simulink model "Lab_1_Part_1_6"  (R2019b)
settings: Solver=VariableStepAuto  StartTime=0.0  StopTime=10.0  RelTol=1e-3
settings Model: Creator=mikewang  LastModifiedBy=mikewang

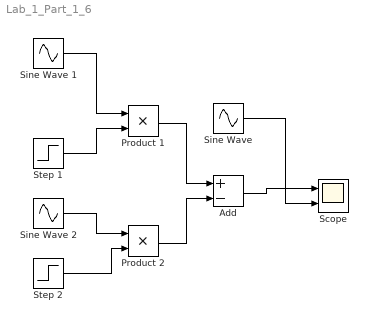
== system Lab_1_Part_1_6 ==
  "Add " : Sum  Inputs=+-
  Product 1 : Product
  Product 2 : Product
  "Scope " : Scope  NumInputPorts=2
  Sine Wave : Sin  Frequency=1000  SampleTime=1e-6
  Sine Wave 1 : Sin  SineType=Sample based  Amplitude=0.5  Samples=1000  SampleTime=0.001
  Sine Wave 2 : Sin  SineType=Sample based  Amplitude=0.5  Samples=1000  SampleTime=0.001
  Step 1 : Step  Time=2  SampleTime=0
  Step 2 : Step  Time=4  SampleTime=0
  wires:
  Sine Wave 1/1 -> Product 1/1
  Step 1/1 -> Product 1/2
  Sine Wave 2/1 -> Product 2/1
  Step 2/1 -> Product 2/2
  Product 1/1 -> "Add "/1
  Product 2/1 -> "Add "/2
  "Add "/1 -> "Scope "/1
  Sine Wave/1 -> "Scope "/2
